simulink model "Non_Linear_Simulator_Jetstar"  (R2020a)
settings: Solver=ode4  StartTime=0.0  StopTime=200  FixedStep=0.01  RelTol=1e-3
libraries: simulink_extras x7, shared6dof x1, vrlib x1
settings Model: OrderedModelArguments=off  Creator=mohan  LastModifiedBy=mohan
settings SolverCC: AlgebraicLoopSolver=LineSearch

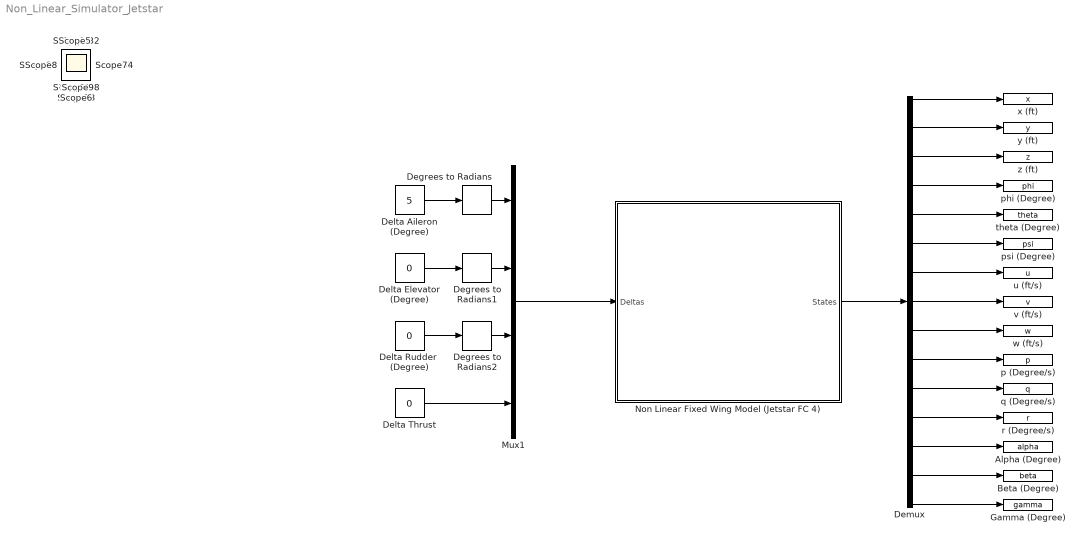
== system Non_Linear_Simulator_Jetstar ==
  Alpha (Degree) : ToWorkspace  VariableName=alpha  SaveFormat=Timeseries  SampleTime=-1
  Beta (Degree) : ToWorkspace  VariableName=beta  SaveFormat=Timeseries  SampleTime=-1
  Degrees to Radians : simulink_extras/Transformations/Degrees to Radians
  Degrees to Radians1 : simulink_extras/Transformations/Degrees to Radians
  Degrees to Radians2 : simulink_extras/Transformations/Degrees to Radians
  Delta Aileron (Degree) : Constant  Value=5
  Delta Elevator (Degree) : Constant  Value=0
  Delta Rudder  (Degree) : Constant  Value=0
  Delta Thrust : Constant  Value=0
  Demux : Demux  Outputs=15
  Gamma (Degree) : ToWorkspace  VariableName=gamma  SaveFormat=Timeseries  SampleTime=-1
  Mux1 : Mux
  Non Linear Fixed Wing Model (Jetstar FC 4) : Subsystem  mask{m=1187.447648, g=32.17405, Ixx=1.19E+05, Iyy=1.36E+05, Izz=2.44E+05, Ixz=5.06E+03, Ixy=0, Iyz=0, L_th=-8.2e-1, VT=586, t0=0, tf=200, h=0.01, Xu=-0.0136, Zu=-0.0305, Mu=0.000727, Xw=0.01, Zw=-1.65, Mw=-0.0201, Zw_dot=0, Zq=0, Mw_dot=-0.000906, Mq=-1.33, Xdel_e=3.51, Zdel_e=-74.5, Mdel_e=-14.6, Xdel_t=8.42e-4, Zdel_t=0, Mdel_t=-6.04e-6, Yv=-2.29e-1, YB=-1.34e2, LB_dash=-7.28, NB_dash=5.47, Lp_dash=-1.75, Np_dash=-1.87e-1, Lr_dash=1.7e-1, Nr_dash=-3.33e-1, Ydel_a_star=0, Ldel_a_dash=5.71, Ndel_a_dash=-5.24e-2, Ydel_r_star=5.57e-2, Ldel_r_dash=2.77, Ndel_r_dash=-3.12, Yp=0, Yr=0, x0=0, y0=0, z0=0, u_0=585.3494667, v_0=0, w_0=27.60438012, p_0=0, q_0=0, r_0=0, udot_0=0, vdot_0=0, wdot_0=0, phai_0=0, theta_0=4.71e-02, psi_0=0}
      mask prompts: m "Mass"; g "Gravity"; L_th "Perpindicular Distance to Thrust Line from C.G"; VT "True Speed (FPS)"; t0 "Start Time"; tf "Stop Time"; h "Time Step"
      mask DialogControl Time Prompt: Time Properties
      mask DialogControl Derivatives Prompt: Aerodynamics Derivatives
      mask DialogControl States Prompt: Initial States
      mask Display: image('$imagefile'); % Use "Edit Image" on toolstrip to change.
  p (Degree/s) : ToWorkspace  VariableName=p  SaveFormat=Timeseries  SampleTime=-1
  phi (Degree) : ToWorkspace  VariableName=phi  SaveFormat=Timeseries  SampleTime=-1
  psi (Degree) : ToWorkspace  VariableName=psi  SaveFormat=Timeseries  SampleTime=-1
  q (Degree/s) : ToWorkspace  VariableName=q  SaveFormat=Timeseries  SampleTime=-1
  r (Degree/s) : ToWorkspace  VariableName=r  SaveFormat=Timeseries  SampleTime=-1
  theta (Degree) : ToWorkspace  VariableName=theta  SaveFormat=Timeseries  SampleTime=-1
  u (ft/s) : ToWorkspace  VariableName=u  SaveFormat=Timeseries  SampleTime=-1
  v (ft/s) : ToWorkspace  VariableName=v  SaveFormat=Timeseries  SampleTime=-1
  w (ft/s) : ToWorkspace  VariableName=w  SaveFormat=Timeseries  SampleTime=-1
  x (ft) : ToWorkspace  VariableName=x  SaveFormat=Timeseries  SampleTime=-1
  y (ft) : ToWorkspace  VariableName=y  SaveFormat=Timeseries  SampleTime=-1
  z (ft) : ToWorkspace  VariableName=z  SaveFormat=Timeseries  SampleTime=-1
  Scope{,1..35} (36 alike) : Scope
  wires:
  Delta Elevator (Degree)/1 -> Degrees to Radians1/1
  Delta Thrust/1 -> Mux1/4
  Delta Aileron (Degree)/1 -> Degrees to Radians/1
  Delta Rudder  (Degree)/1 -> Degrees to Radians2/1
  Mux1/1 -> Non Linear Fixed Wing Model (Jetstar FC 4)/1(Deltas)
  Non Linear Fixed Wing Model (Jetstar FC 4)/1(States) -> Demux/1
  Demux/1 -> x (ft)/1
  Demux/2 -> y (ft)/1
  Demux/3 -> z (ft)/1
  Demux/5 -> theta (Degree)/1
  Demux/7 -> u (ft/s)/1
  Demux/8 -> v (ft/s)/1
  Demux/9 -> w (ft/s)/1
  Demux/10 -> p (Degree/s)/1
  Demux/11 -> q (Degree/s)/1
  Demux/12 -> r (Degree/s)/1
  Demux/13 -> Alpha (Degree)/1
  Demux/14 -> Beta (Degree)/1
  Degrees to Radians/1 -> Mux1/1
  Degrees to Radians1/1 -> Mux1/2
  Degrees to Radians2/1 -> Mux1/3
  Demux/4 -> phi (Degree)/1
  Demux/6 -> psi (Degree)/1
  Demux/15 -> Gamma (Degree)/1

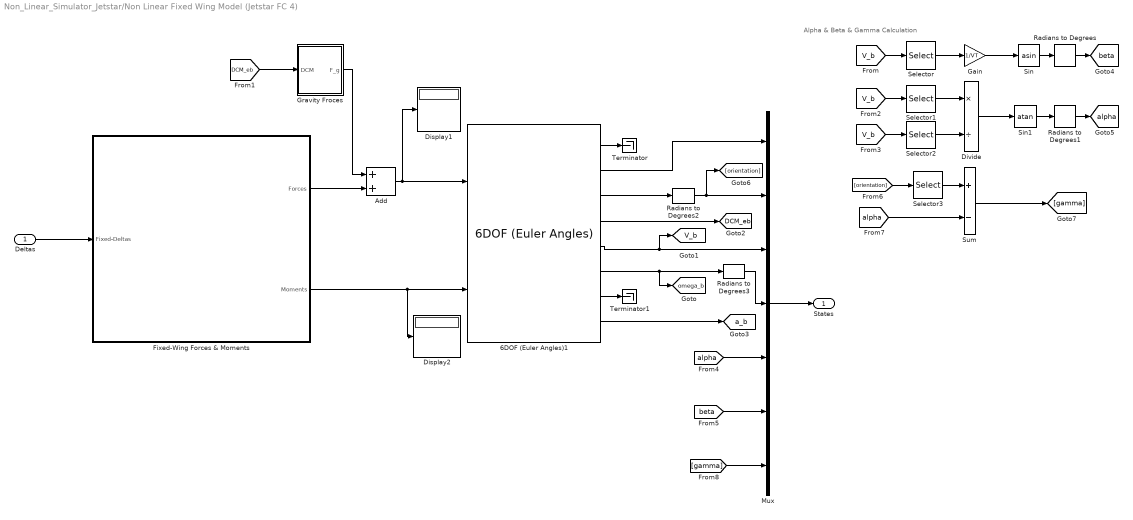
== system Non_Linear_Simulator_Jetstar/Non Linear Fixed Wing Model (Jetstar FC 4) ==
  note: Alpha & Beta & Gamma Calculation
  Deltas : Inport
  6DOF (Euler Angles)1 : shared6dof/6DOF (Euler Angles)  units=English (Velocity in ft/s)  mtype=Fixed  rep=Euler Angles  xme_0=[x0 y0 z0]  Vm_0=[u_0 v_0 w_0]  eul_0=[phai_0 theta_0 psi_0]  pm_0=[p_0 q_0 r_0]  mass_0=m  mass_e=0.5  mass_f=2.0  inertia=[Ixx -Ixy -Ixz ; -Ixy Iyy -Iyz ; -Ixz -Iyz Izz]  inertia_e=eye(3)  inertia_f=2*eye(3)  k_quat=1.0  vre_flag=on  abi_flag=off  aMode=aMode  xme_statename=''  Vm_statename=''  eul_statename=''  quat_statename=''  pm_statename=''  mass_statename=''
      settings: SourceProductBaseCode=AE,PW,MT,VE,VP
  Add : Sum  Inputs=2
  Display1 : Display
  Display2 : Display
  Divide : Product  Inputs=*/
  Fixed-Wing Forces & Moments : Subsystem
  Gain : Gain  Gain=1/VT
  Gravity Froces : Subsystem
  Mux : Mux  Inputs=7
  Radians to Degrees{,1..3} (4 alike) : simulink_extras/Transformations/Radians to Degrees
  Selector : Selector  InputPortWidth=3  IndexOptions=Starting index (dialog)  Indices=2  OutputSizes=1
  Selector1 : Selector  InputPortWidth=3  IndexOptions=Starting index (dialog)  Indices=3  OutputSizes=1
  Selector2 : Selector  InputPortWidth=3  IndexOptions=Starting index (dialog)  Indices=1  OutputSizes=1
  Selector3 : Selector  InputPortWidth=3  IndexOptions=Starting index (dialog)  Indices=2  OutputSizes=1
  Sin : Trigonometry  Operator=asin
  Sin1 : Trigonometry  Operator=atan
  Sum : Sum  Inputs=+-
  Terminator : Terminator
  Terminator1 : Terminator
  States : Outport
  tag scope: DCM_eb=global, V_b=global, a_b=global, alpha=global, beta=global, omega_b=global
  wires:
  Gravity Froces/1(F_g) -> Add/1
  6DOF (Euler Angles)1/2 -> Mux/1
  6DOF (Euler Angles)1/1 -> Terminator/1
  Mux/1 -> States/1
  6DOF (Euler Angles)1/7 -> Terminator1/1
  Fixed-Wing Forces & Moments/1(Forces) -> Add/2
  Add/1 -> 6DOF (Euler Angles)1/1, Display1/1
  Fixed-Wing Forces & Moments/2("Moments ") -> Display2/1, 6DOF (Euler Angles)1/2
  6DOF (Euler Angles)1/4 -> [DCM_eb]
  6DOF (Euler Angles)1/8 -> [a_b]
  [DCM_eb] -> Gravity Froces/1(DCM)
  [V_b] -> Selector/1
  Selector/1 -> Gain/1
  Gain/1 -> Sin/1
  Sin/1 -> Radians to Degrees/1
  Divide/1 -> Sin1/1
  Selector1/1 -> Divide/1
  Sin1/1 -> Radians to Degrees1/1
  [V_b] -> Selector1/1
  [V_b] -> Selector2/1
  Selector2/1 -> Divide/2
  [alpha] -> Mux/5
  [beta] -> Mux/6
  Radians to Degrees/1 -> [beta]
  Radians to Degrees1/1 -> [alpha]
  6DOF (Euler Angles)1/3 -> Radians to Degrees2/1
  6DOF (Euler Angles)1/6 -> [omega_b], Radians to Degrees3/1
  Deltas/1 -> Fixed-Wing Forces & Moments/1(Fixed-Deltas)
  Radians to Degrees2/1 -> [orientation], Mux/2
  6DOF (Euler Angles)1/5 -> [V_b], Mux/3
  Radians to Degrees3/1 -> Mux/4
  [alpha] -> Sum/2
  Selector3/1 -> Sum/1
  [orientation] -> Selector3/1
  Sum/1 -> [gamma]
  [gamma] -> Mux/7

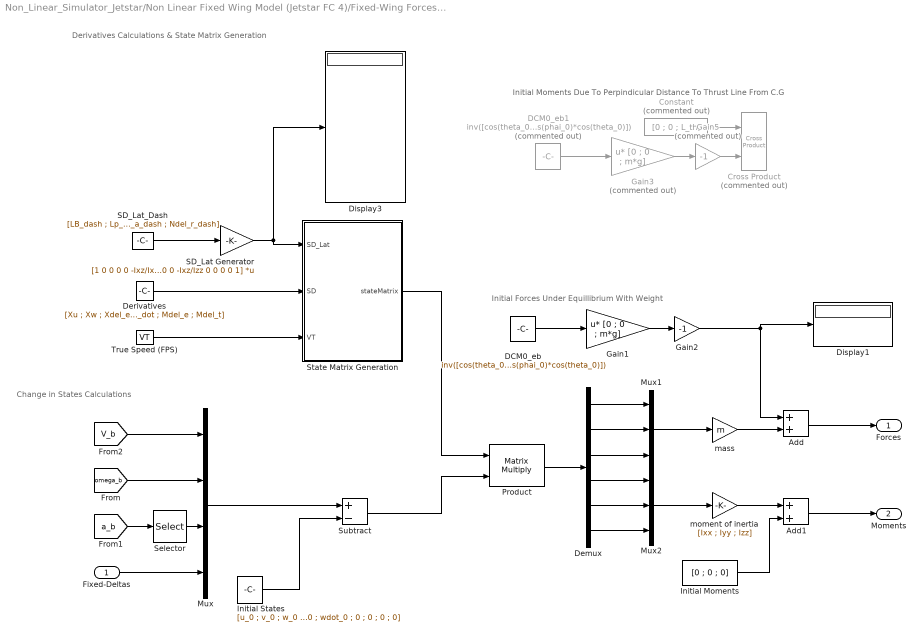
== system Non_Linear_Simulator_Jetstar/Non Linear Fixed Wing Model (Jetstar FC 4)/Fixed-Wing Forces & Moments ==
  note: Change in States Calculations
  note: Derivatives Calculations & State Matrix Generation
  note: Initial Forces Under Equillibrium With Weight
  note: Initial Moments Due To Perpindicular Distance To Thrust Line From C.G
  Fixed-Deltas : Inport
  Add : Sum
  Add1 : Sum
  Constant : Constant  Commented=on  Value=[0 ; 0 ; L_th]
  Cross Product : vrlib/Utilities/Cross Product  Commented=on
  DCM0_eb : Constant  Value="inv([cos(theta_0)*cos(psi_0) , (sin(phai_0)*sin(theta_0)*cos(psi_0)-cos(phai_0)*sin(psi_0)) , (cos(phai_0)*sin(theta_0)*cos(psi_0)+sin(phai_0)*sin(psi_0)) ; cos(theta_0)*sin(psi_0) , (sin(phai_0)*sin(theta_0)*sin(psi_0)+cos(phai_0)*cos(psi_0)) , (cos(phai_0)*sin(theta_0)*sin(psi_0)-sin(phai_0)*cos(psi_0)) ;  -sin(theta_0) ,  sin(phai_0)*cos(theta_0)  , cos(phai_0)*cos(theta_0)])"
  DCM0_eb1 : Constant  Commented=on  Value="inv([cos(theta_0)*cos(psi_0) , (sin(phai_0)*sin(theta_0)*cos(psi_0)-cos(phai_0)*sin(psi_0)) , (cos(phai_0)*sin(theta_0)*cos(psi_0)+sin(phai_0)*sin(psi_0)) ; cos(theta_0)*sin(psi_0) , (sin(phai_0)*sin(theta_0)*sin(psi_0)+cos(phai_0)*cos(psi_0)) , (cos(phai_0)*sin(theta_0)*sin(psi_0)-sin(phai_0)*cos(psi_0)) ;  -sin(theta_0) ,  sin(phai_0)*cos(theta_0)  , cos(phai_0)*cos(theta_0)])"
  Demux : Demux  Outputs=6
  Derivatives : Constant  Value=[Xu ; Xw ; Xdel_e ; Xdel_t ; Yv ; Yp ; Yr ; Ydel_r_star ; Zu ; Zw ; Zq ; Zw_dot ; Zdel_e ; Zdel_t ; Mu ; Mw ; Mq ; Mw_dot ; Mdel_e ; Mdel_t]
  Display1 : Display
      settings: Decimation=4
  Display3 : Display
  Gain1 : Gain  Gain=[0 ; 0 ; m*g]  Multiplication=Matrix(u*K)
  Gain2 : Gain  Gain=-1
  Gain3 : Gain  Commented=on  Gain=[0 ; 0 ; m*g]  Multiplication=Matrix(u*K)
  Gain5 : Gain  Commented=on  Gain=-1
  Initial Moments : Constant  Value=[0 ; 0 ; 0]
  Initial States : Constant  Value=[u_0 ; v_0 ; w_0 ; p_0 ; q_0 ; r_0 ; wdot_0 ; 0 ; 0 ; 0 ; 0]
  Mux : Mux
  Mux1 : Mux  Inputs=3
  Mux2 : Mux  Inputs=3
  Product : Product  Multiplication=Matrix(*)
  SD_Lat Generator : Gain  Gain="[1 0 0 0 0 -Ixz/Ixx 0 0 0 0 ; 0 1 0 0 0 0 -Ixz/Ixx 0 0 0 ; 0 0 1 0 0 0 0 -Ixz/Ixx 0  0 ; 0 0 0 1 0 0 0 0 -Ixz/Ixx 0 ; 0 0 0 0 1 0 0 0 0 -Ixz/Ixx ; -Ixz/Izz 0 0 0 0 1 0 0 0 0 ; 0 -Ixz/Izz 0 0 0 0 1 0 0 0 ; 0 0 -Ixz/Izz 0 0 0 0 1 0 0 ; 0 0 0 -Ixz/Izz 0 0 0 0 1 0 ;  0 0 0 0 -Ixz/Izz 0 0 0 0 1]"  Multiplication=Matrix(K*u)
  SD_Lat_Dash : Constant  Value=[LB_dash ; Lp_dash ; Lr_dash ; Ldel_a_dash ; Ldel_r_dash ; NB_dash ; Np_dash ; Nr_dash ; Ndel_a_dash ; Ndel_r_dash]
  Selector : Selector  InputPortWidth=3  IndexOptions=Starting index (dialog)  Indices=3  OutputSizes=1
  State Matrix Generation : MATLAB Function  TreatAsAtomicUnit=on
  Subtract : Sum  Inputs=+-
  True Speed (FPS) : Constant  Value=VT
  mass : Gain  Gain=m
  moment of inertia : Gain  Gain=[Ixx ; Iyy ; Izz]
  Forces : Outport
  "Moments " : Outport  Port=2
  wires:
  Selector/1 -> Mux/3
  Fixed-Deltas/1 -> Mux/4
  [omega_b] -> Mux/2
  [V_b] -> Mux/1
  Mux/1 -> Subtract/1
  Subtract/1 -> Product/2
  Initial States/1 -> Subtract/2
  Demux/2 -> Mux1/2
  Demux/1 -> Mux1/1
  Demux/3 -> Mux1/3
  Demux/4 -> Mux2/1
  Demux/5 -> Mux2/2
  Demux/6 -> Mux2/3
  Mux1/1 -> mass/1
  Mux2/1 -> moment of inertia/1
  mass/1 -> Add/2
  moment of inertia/1 -> Add1/1
  Add/1 -> Forces/1
  Add1/1 -> "Moments "/1
  DCM0_eb/1 -> Gain1/1
  Gain1/1 -> Gain2/1
  Gain2/1 -> Add/1, Display1/1
  Gain3/1 -> Gain5/1
  DCM0_eb1/1 -> Gain3/1
  Gain5/1 -> Cross Product/2
  Constant/1 -> Cross Product/1
  Initial Moments/1 -> Add1/2
  SD_Lat_Dash/1 -> SD_Lat Generator/1
  SD_Lat Generator/1 -> Display3/1, State Matrix Generation/1(SD_Lat)
  Product/1 -> Demux/1
  State Matrix Generation/1(stateMatrix) -> Product/1
  Derivatives/1 -> State Matrix Generation/2(SD)
  True Speed (FPS)/1 -> State Matrix Generation/3(VT)
  [a_b] -> Selector/1

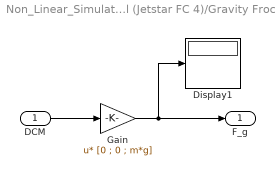
== system Non_Linear_Simulator_Jetstar/Non Linear Fixed Wing Model (Jetstar FC 4)/Gravity Froces ==
  DCM : Inport
  Display1 : Display
  Gain : Gain  Gain=[0 ; 0 ; m*g]  Multiplication=Matrix(u*K)
  F_g : Outport
  wires:
  Gain/1 -> F_g/1, Display1/1
  DCM/1 -> Gain/1

== matlab function Non_Linear_Simulator_Jetstar/Non Linear Fixed Wing Model (Jetstar FC 4)/Fixed-Wing Forces & Moments/State Matrix Generation ==
  data: SD_Lat input; stateMatrix output; SD input; VT input
function stateMatrix = stateMatrixGenerator(SD_Lat,SD,VT)
stateMatrix=zeros(6,11);

Xu=SD(1);   Xw=SD(2);       Xdel_e=SD(3);       Xdel_t=SD(4);   Yv=SD(5);
Yp=SD(6);   Yr=SD(7);       Ydel_r_star=SD(8);  Zu=SD(9);       Zw=SD(10);
Zq=SD(11);  Zw_dot=SD(12);  Zdel_e=SD(13);      Zdel_t=SD(14);   Mu=SD(15); 
Mw=SD(16);  Mq=SD(17);      Mw_dot=SD(18);      Mdel_e=SD(19);   Mdel_t=SD(20);

LB=SD_Lat(1);   Lp=SD_Lat(2);   Lr=SD_Lat(3);   Ldel_a=SD_Lat(4);
Ldel_r=SD_Lat(5);
NB=SD_Lat(6);   Np=SD_Lat(7);   Nr=SD_Lat(8);   Ndel_a=SD_Lat(9);   
Ndel_r=SD_Lat(10);

Ydel_r=Ydel_r_star*VT;
Lv=LB/VT;
Nv=NB/VT;

stateMatrix=...
     [Xu ,   0 ,     Xw ,    0 ,     0 ,     0 ,     0 ,     0 ,     Xdel_e ,    0 ,     Xdel_t ; 
      0 ,   Yv ,    0 ,     Yp ,    0 ,     Yr ,     0 ,    0 ,     0 ,     Ydel_r ,        0 ; 
      Zu ,  0 ,     Zw ,     0 ,     Zq ,    0 ,     Zw_dot , 0   , Zdel_e , 0 ,         Zdel_t ; 
      0 ,   Lv ,    0 ,      Lp ,    0 ,     Lr ,     0 ,   Ldel_a , 0 ,     Ldel_r ,    0 ; 
      Mu , 0 , Mw , 0 , Mq , 0 , Mw_dot , 0 , Mdel_e , 0 , Mdel_t ; 
      0 , Nv , 0 , Np , 0 , Nr , 0 , Ndel_a , 0 , Ndel_r ,                                  0];
end
